simulink library "Lib_LongPRACH"  (R2023b)
settings: Solver=VariableStepAuto  StartTime=0.0  StopTime=10.0  RelTol=1e-3
values from neighbouring files (symbols this model uses):
  prach = waveconfig.PRACH.Config    [hNRPRACHWaveformGenerator.m]
undefined symbols (not defined in the file or in its folder): AdvDSPBChannelOutDisplay, AdvDSPBDMemDisplay, AdvDSPBInDisplay, AdvDSPBOutDisplay, dpoly, dspba, dspba_ChannelInVis, dspba_ChannelOutVis, dspba_internal_get_channel_ports, evalAionMaskParam, latency, latencyCorrection, NTxAnts, primtype, UseDontCare, value
libraries: DSPBAPrim x553, DSPBABase x32, DSPBAFilters x24, DSPBAControl x18, DSPBAModelBus x8, DSPBAWaveformSynth x4, DspbAdvFftLibrary x2, DSPBAUtilities x2
(part 1 of 8)
settings Model: Creator=manjukri  LastModifiedBy=5g
settings ModelReferenceCC: EnableRefExpFcnMdlSchedulingChecks=on

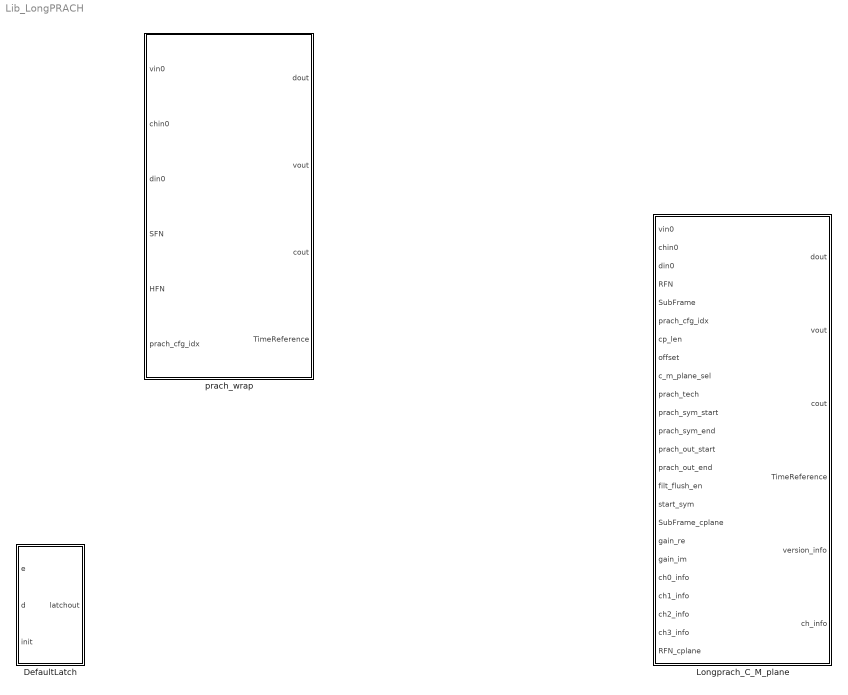
== system Lib_LongPRACH ==
  DefaultLatch : Subsystem
  Longprach_C_M_plane : Subsystem  mask{AxCdelay=60, FFT_frac_scaling=8, gain_out_frac=11}
      mask prompts: AxCdelay "Enter the output delay between antenna(min 60)"; FFT_frac_scaling "FFT output Fractional bits"; gain_out_frac "Gain block output fractional bits"
      mask init:
      | fsmpaths
      | %% 3GPP TS 38.211 V17.2  Table 6.3.3.2-3
      | 
      | Map_5g_LUT1 = [9 9 9 9 9 4 4 9 8 7 6 5 4 3 2 1 1 4 3 2 8 4 3 7 3 6 1 1 zeros(1,512-35) 7 7 7 7 7 2 2 ];
      | Map_5g_LUT2 = [9 9 9 9 9 4 4 9 8 7 6 5 4 3 2 6 6 9 8 7 9 8 4 8 4 7 4 3 zeros(1,512-35) 7 7 7 7 7 2 2 ];
      | Map_5g_LUT3 = [9 9 9 9 9 4 4 9 8 7 6 5 4 3 2 6 6 9 8 7 9 9 9 9 8 8 6 5 zeros(1,512-35) 7 7 7 7 7 2 2 ];
      | Map_5g_LUT4 = [9 9 9 9 9 4 4 9 8 7 6 5 4 3 2 6 6 9 8 7 9 9 9 9 9 9 9 7 zeros(1,512-35) 7 7 7 7 7 2 2 ];
      | Map_5g_LUT5 = [9 9 9 9 9 4 4 9 8 7 6 5 4 3 2 6 6 9 8 7 9 9 9 9 9 9 9 9 zeros(1,512-35) 7 7 7 7 7 2 2 ];
      | 
      | 
      | x_lut = [16,8,4,2,2,2,2,ones(1,512-14),16,8,4,2,2,2,2];
      | y_lut = [1 1 1 0 1 0  1 zeros(1,512-14) 1 1 1 0 1 0 1];
      | 
      | startsym_lut=[ones(1,16) 8 ones(1,512-17)];
  prach_wrap : Subsystem  mask{LongFormat=0, prach_technology=1, AxCdelay=60, PRACH_SCS=1.25, FFT_frac_scaling=12}
      mask prompts: LongFormat "Enter PRACH Long Format"; prach_technology "Enter Technology : 0=4G , 1=5G"; AxCdelay "Enter the output delay between antenna(min 60)"; PRACH_SCS "Enter PRACH subcarrier Spacing (KHz)"; FFT_frac_scaling "FFT output Fractional bits"
      mask init:
      | fsmpaths
      | %% 3GPP TS 38.211 V17.2  Table 6.3.3.2-3
      | 
      | Map_5g_LUT1 = [9 9 9 9 9 4 4 9 8 7 6 5 4 3 2 1 1 4 3 2 8 4 3 7 3 6 1 1 zeros(1,256-28)];
      | Map_5g_LUT2 = [9 9 9 9 9 4 4 9 8 7 6 5 4 3 2 6 6 9 8 7 9 8 4 8 4 7 4 3 zeros(1,256-28)];
      | Map_5g_LUT3 = [9 9 9 9 9 4 4 9 8 7 6 5 4 3 2 6 6 9 8 7 9 9 9 9 8 8 6 5 zeros(1,256-28)];
      | Map_5g_LUT4 = [9 9 9 9 9 4 4 9 8 7 6 5 4 3 2 6 6 9 8 7 9 9 9 9 9 9 9 7 zeros(1,256-28)];
      | Map_5g_LUT5 = [9 9 9 9 9 4 4 9 8 7 6 5 4 3 2 6 6 9 8 7 9 9 9 9 9 9 9 9 zeros(1,256-28)];

== system Lib_LongPRACH/DefaultLatch ==
  e : Inport
  d : Inport  Port=2
  init : Inport  Port=3
  Mux : DSPBAPrim/Mux  primtype=mux  nInputs=evalAionMaskParam(gcb,'value',1)+1  nOutputs=1  omode=Inherit via internal rule  otype=sfix(16)  scale=2^-15  rndmethod=Unbiased  factor=1  satmethod=Symmetric  shift_vec=[0 1 2 -1]  value=2  inPortNames=['s '; 'd0'; 'd1'; 'd2'; 'd3'; 'd4'; 'd5'; 'd6'; 'd7'; 'd8'; 'd9';]  outPortNames=[' ']  dspbaimage=dspba_prim_tall.svg  text=fprintf('%s', primtype);  style=Optimised  visibilities=1032  version=20211007
  Or : DSPBAPrim/Or  primtype=or  nInputs=2  nOutputs=1  omode=Inherit via internal rule  otype=sfix(16)  scale=2^-15  rndmethod=Unbiased  factor=1  satmethod=Symmetric  shift_vec=[0 1 2 -1]  value=0  inPortNames=[' '; ' '; ' '; ' '; ' '; ' '; ' '; ' '; ' '; ' '; ' '; ' '; ' '; ' '; ' '; ' '; ]  outPortNames=[' ']  dspbaimage=dspba_prim.svg  text=fprintf('|');  style=Optimised  visibilities=8+2  version=20211007
  SampleDelay : DSPBAPrim/SampleDelay  primtype=sampdelay  nInputs=1  nOutputs=1  omode=Inherit via internal rule  otype=sfix(16)  scale=2^-15  rndmethod=Unbiased  factor=1  satmethod=Symmetric  shift_vec=[0 1 2 -1]  floatPrecision=float32_m23  value=1  inPortNames=[' '; ' ';]  outPortNames=[' ']  dspbaimage=dspba_prim.svg  text=dpoly(1, eye(1,value+1), 'z')  style=Optimised  visibilities=8 + 2^11 + 2^18 + 2^19  flexible=off  slackgroup=0  augmented=0  version=20211007  advOptions=[]
  latch_0L : DSPBAControl/latch_0L
  latchout : Outport
  wires:
  Or/1 -> SampleDelay/1, Mux/1
  Mux/1 -> latchout/1
  e/1 -> latch_0L/1, Or/1
  SampleDelay/1 -> Or/2
  init/1 -> Mux/2
  latch_0L/1 -> Mux/3
  d/1 -> latch_0L/2

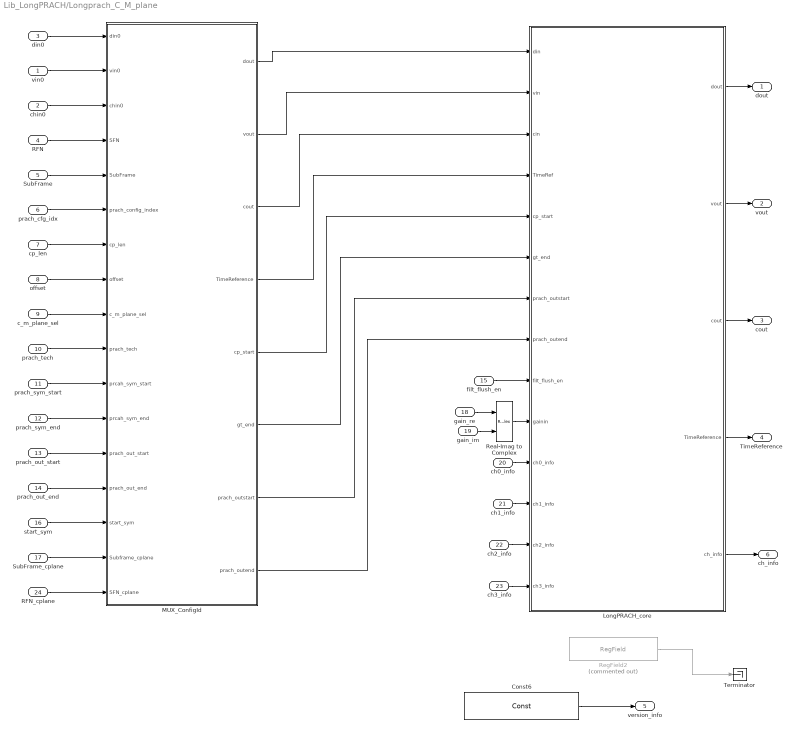
== system Lib_LongPRACH/Longprach_C_M_plane ==
  vin0 : Inport
  chin0 : Inport  Port=2
  din0 : Inport  Port=3
  RFN : Inport  Port=4
  SubFrame : Inport  Port=5
  prach_cfg_idx : Inport  Port=6
  cp_len : Inport  Port=7
  offset : Inport  Port=8
  c_m_plane_sel : Inport  Port=9
  prach_tech : Inport  Port=10
  prach_sym_start : Inport  Port=11
  prach_sym_end : Inport  Port=12
  prach_out_start : Inport  Port=13
  prach_out_end : Inport  Port=14
  filt_flush_en : Inport  Port=15
  start_sym : Inport  Port=16
  SubFrame_cplane : Inport  Port=17
  gain_re : Inport  Port=18
  gain_im : Inport  Port=19
  ch0_info : Inport  Port=20
  ch1_info : Inport  Port=21
  ch2_info : Inport  Port=22
  ch3_info : Inport  Port=23
  RFN_cplane : Inport  Port=24
  Const6 : DSPBAPrim/Const  primtype=const  nInputs=0  nOutputs=1  omode=Specify via dialog  otype=ufix(32)  scale=2^0  rndmethod=Unbiased  factor=1  satmethod=Symmetric  shift_vec=[0 1 2 -1]  value=Version_reg_val  inPortNames=['+'; '+';]  outPortNames=[' ']  dspbaimage=dspba_prim.svg  text=fprintf('%s', num2str(value));  style=Optimised  visibilities=8 + 1024  floatPrecision=float32_m23  warnSaturation=on  version=20211007  SampleTime=inf
  LongPRACH_core : Subsystem
  MUX_ConfigId : Subsystem
  Real-Imag to Complex : RealImagToComplex
  RegField2 : DSPBAModelBus/RegField  Commented=on  reg_name=MMoffset.versionreg  reg_rwmode=Constant  reg_msb=31  reg_lsb=0  reg_mode=Specify via dialog  reg_type=ufix(32)  reg_scale=2^0  reg_init=Version_reg_val  reg_desc=version register  reg_modal=off  reg_desc0=0  reg_desc1=0  reg_desc2=0  reg_desc3=0  reg_desc4=0  reg_desc5=0  reg_desc6=0  reg_desc7=0  reg_addr=4  SampleTime=-1  version=20090407
  Terminator : Terminator
  dout : Outport  VectorParamsAs1DForOutWhenUnconnected=off
  vout : Outport  Port=2  VectorParamsAs1DForOutWhenUnconnected=off
  cout : Outport  Port=3  VectorParamsAs1DForOutWhenUnconnected=off
  TimeReference : Outport  Port=4  VectorParamsAs1DForOutWhenUnconnected=off
  version_info : Outport  Port=5
  ch_info : Outport  Port=6
  wires:
  MUX_ConfigId/7(prach_outstart) -> LongPRACH_core/7(prach_outstart)
  MUX_ConfigId/8(prach_outend) -> LongPRACH_core/8(prach_outend)
  MUX_ConfigId/2(vout) -> LongPRACH_core/2(vin)
  start_sym/1 -> MUX_ConfigId/15(start_sym)
  din0/1 -> MUX_ConfigId/1(din0)
  prach_out_end/1 -> MUX_ConfigId/14(prach_out_end)
  MUX_ConfigId/1(dout) -> LongPRACH_core/1(din)
  prach_out_start/1 -> MUX_ConfigId/13(prach_out_start)
  prach_cfg_idx/1 -> MUX_ConfigId/6(prach_config_index)
  MUX_ConfigId/6(gt_end) -> LongPRACH_core/6(gt_end)
  c_m_plane_sel/1 -> MUX_ConfigId/9(c_m_plane_sel)
  LongPRACH_core/4(TimeReference) -> TimeReference/1
  chin0/1 -> MUX_ConfigId/3(chin0)
  filt_flush_en/1 -> LongPRACH_core/9(filt_flush_en)
  LongPRACH_core/3(cout) -> cout/1
  prach_sym_start/1 -> MUX_ConfigId/11(prcah_sym_start)
  LongPRACH_core/1(dout) -> dout/1
  SubFrame/1 -> MUX_ConfigId/5(SubFrame)
  RFN/1 -> MUX_ConfigId/4(SFN)
  vin0/1 -> MUX_ConfigId/2(vin0)
  LongPRACH_core/2(vout) -> vout/1
  MUX_ConfigId/5(cp_start) -> LongPRACH_core/5(cp_start)
  prach_tech/1 -> MUX_ConfigId/10(prach_tech)
  SubFrame_cplane/1 -> MUX_ConfigId/16(Subframe_cplane)
  MUX_ConfigId/3(cout) -> LongPRACH_core/3(cin)
  MUX_ConfigId/4(TimeReference) -> LongPRACH_core/4(TimeRef)
  offset/1 -> MUX_ConfigId/8(offset)
  prach_sym_end/1 -> MUX_ConfigId/12(prcah_sym_end)
  cp_len/1 -> MUX_ConfigId/7(cp_len)
  Real-Imag to Complex/1 -> LongPRACH_core/10(gainin)
  gain_re/1 -> Real-Imag to Complex/1
  gain_im/1 -> Real-Imag to Complex/2
  RegField2/1 -> Terminator/1
  Const6/1 -> version_info/1
  ch0_info/1 -> LongPRACH_core/11(ch0_info)
  ch2_info/1 -> LongPRACH_core/13(ch2_info)
  ch1_info/1 -> LongPRACH_core/12(ch1_info)
  ch3_info/1 -> LongPRACH_core/14(ch3_info)
  LongPRACH_core/5(ch_info) -> ch_info/1
  RFN_cplane/1 -> MUX_ConfigId/17(SFN_cplane)

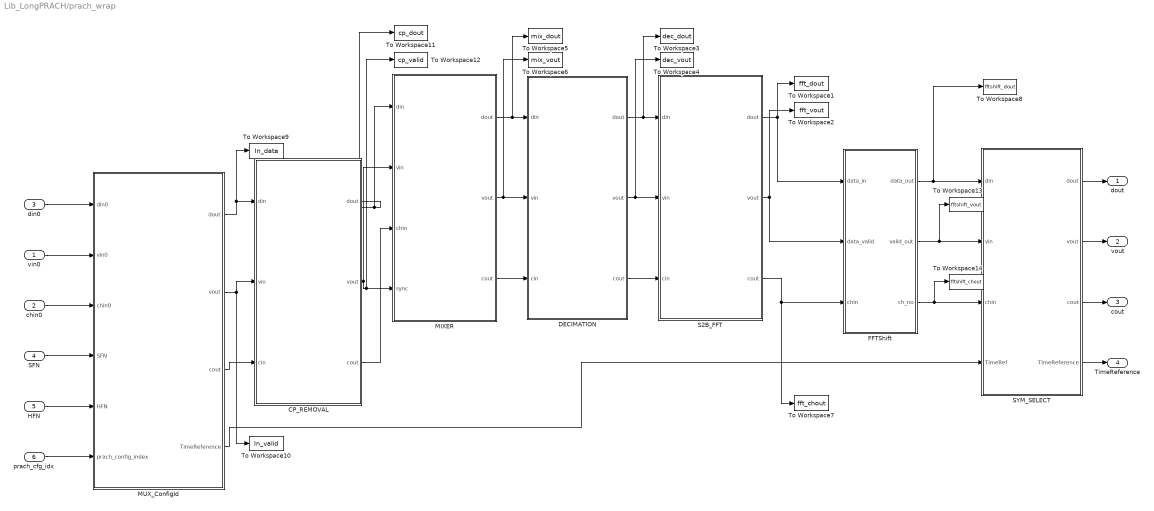
== system Lib_LongPRACH/prach_wrap ==
  vin0 : Inport
  chin0 : Inport  Port=2
  din0 : Inport  Port=3
  SFN : Inport  Port=4
  HFN : Inport  Port=5
  prach_cfg_idx : Inport  Port=6
  CP_REMOVAL : Subsystem
  DECIMATION : Subsystem
  FFTShift : Subsystem
  MIXER : Subsystem
  MUX_ConfigId : Subsystem
  S2B_FFT : Subsystem
  SYM_SELECT : Subsystem
  To Workspace1 : ToWorkspace  VariableName=fft_dout  SampleTime=-1
  To Workspace10 : ToWorkspace  VariableName=In_valid  SampleTime=-1
  To Workspace11 : ToWorkspace  VariableName=cp_dout  SampleTime=-1
  To Workspace12 : ToWorkspace  VariableName=cp_valid  SampleTime=-1
  To Workspace13 : ToWorkspace  VariableName=fftshift_vout  SampleTime=-1
  To Workspace14 : ToWorkspace  VariableName=fftshift_chout  SampleTime=-1
  To Workspace2 : ToWorkspace  VariableName=fft_vout  SampleTime=-1
  To Workspace3 : ToWorkspace  VariableName=dec_dout  SampleTime=-1
  To Workspace4 : ToWorkspace  VariableName=dec_vout  SampleTime=-1
  To Workspace5 : ToWorkspace  VariableName=mix_dout  SampleTime=-1
  To Workspace6 : ToWorkspace  VariableName=mix_vout  SampleTime=-1
  To Workspace7 : ToWorkspace  VariableName=fft_chout  SampleTime=-1
  To Workspace8 : ToWorkspace  VariableName=fftshift_dout  SampleTime=-1
  To Workspace9 : ToWorkspace  VariableName=In_data  SampleTime=-1
  dout : Outport  VectorParamsAs1DForOutWhenUnconnected=off
  vout : Outport  Port=2  VectorParamsAs1DForOutWhenUnconnected=off
  cout : Outport  Port=3  VectorParamsAs1DForOutWhenUnconnected=off
  TimeReference : Outport  Port=4  VectorParamsAs1DForOutWhenUnconnected=off
  wires:
  MUX_ConfigId/1(dout) -> To Workspace9/1, CP_REMOVAL/1(din)
  DECIMATION/1(dout) -> S2B_FFT/1(din), To Workspace3/1
  MIXER/2(vout) -> DECIMATION/2(vin), To Workspace6/1
  MUX_ConfigId/2(vout) -> To Workspace10/1, CP_REMOVAL/2(vin)
  CP_REMOVAL/2(vout) -> To Workspace12/1, MIXER/4(sync), MIXER/2(vin)
  MUX_ConfigId/4(TimeReference) -> SYM_SELECT/4(TimeRef)
  S2B_FFT/3(cout) -> FFTShift/3(chin), To Workspace7/1
  DECIMATION/2(vout) -> S2B_FFT/2(vin), To Workspace4/1
  SYM_SELECT/2(vout) -> vout/1
  S2B_FFT/2(vout) -> FFTShift/2(data_valid), To Workspace2/1
  MIXER/3(cout) -> DECIMATION/3(cin)
  CP_REMOVAL/1(dout) -> To Workspace11/1, MIXER/1(din)
  CP_REMOVAL/3(cout) -> MIXER/3(chin)
  MIXER/1(dout) -> DECIMATION/1(din), To Workspace5/1
  DECIMATION/3(cout) -> S2B_FFT/3(cin)
  SYM_SELECT/3(cout) -> cout/1
  SFN/1 -> MUX_ConfigId/4(SFN)
  HFN/1 -> MUX_ConfigId/5(HFN)
  MUX_ConfigId/3(cout) -> CP_REMOVAL/3(cin)
  din0/1 -> MUX_ConfigId/1(din0)
  prach_cfg_idx/1 -> MUX_ConfigId/6(prach_config_index)
  chin0/1 -> MUX_ConfigId/3(chin0)
  S2B_FFT/1(dout) -> FFTShift/1(data_in), To Workspace1/1
  SYM_SELECT/1(dout) -> dout/1
  SYM_SELECT/4(TimeReference) -> TimeReference/1
  vin0/1 -> MUX_ConfigId/2(vin0)
  FFTShift/1(data_out) -> To Workspace8/1, SYM_SELECT/1(din)
  FFTShift/2(valid_out) -> To Workspace13/1, SYM_SELECT/2(vin)
  FFTShift/3(ch_no) -> To Workspace14/1, SYM_SELECT/3(chin)

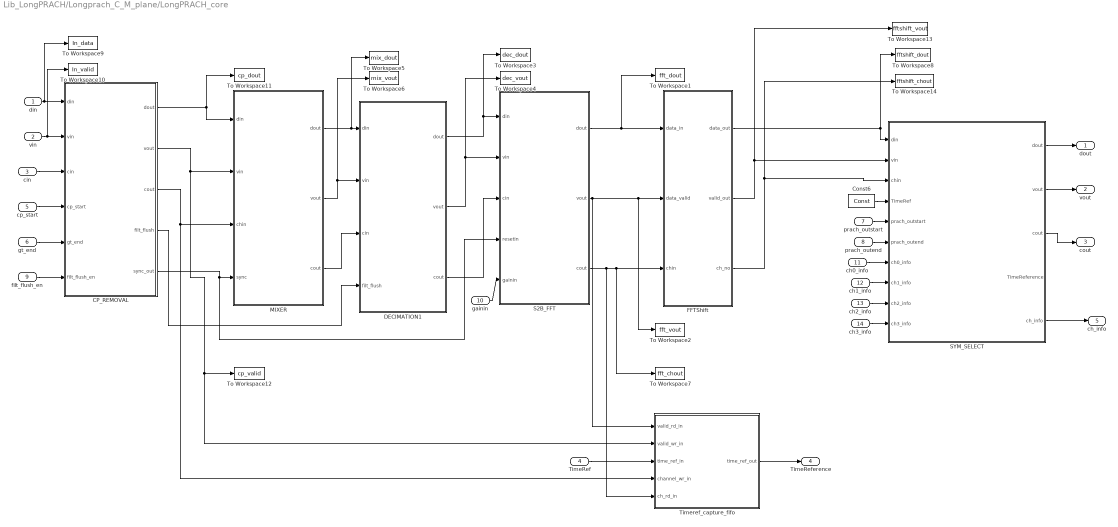
== system Lib_LongPRACH/Longprach_C_M_plane/LongPRACH_core ==
  din : Inport
  vin : Inport  Port=2
  cin : Inport  Port=3
  TimeRef : Inport  Port=4
  cp_start : Inport  Port=5
  gt_end : Inport  Port=6
  prach_outstart : Inport  Port=7
  prach_outend : Inport  Port=8
  filt_flush_en : Inport  Port=9
  gainin : Inport  Port=10
  ch0_info : Inport  Port=11
  ch1_info : Inport  Port=12
  ch2_info : Inport  Port=13
  ch3_info : Inport  Port=14
  CP_REMOVAL : Subsystem
  Const6 : DSPBAPrim/Const  primtype=const  nInputs=0  nOutputs=1  omode=Specify via dialog  otype=ufix(1)  scale=2^0  rndmethod=Unbiased  factor=1  satmethod=Symmetric  shift_vec=[0 1 2 -1]  value=0  inPortNames=['+'; '+';]  outPortNames=[' ']  dspbaimage=dspba_prim.svg  text=fprintf('%s', num2str(value));  style=Optimised  visibilities=8 + 1024  floatPrecision=float32_m23  warnSaturation=on  version=20211007  SampleTime=inf
  DECIMATION1 : Subsystem
  FFTShift : Subsystem
  MIXER : Subsystem
  S2B_FFT : Subsystem
  SYM_SELECT : Subsystem
  Timeref_capture_fifo : Subsystem
  To Workspace1 : ToWorkspace  VariableName=fft_dout  SampleTime=-1
  To Workspace10 : ToWorkspace  VariableName=In_valid  SampleTime=-1
  To Workspace11 : ToWorkspace  VariableName=cp_dout  SampleTime=-1
  To Workspace12 : ToWorkspace  VariableName=cp_valid  SampleTime=-1
  To Workspace13 : ToWorkspace  VariableName=fftshift_vout  SampleTime=-1
  To Workspace14 : ToWorkspace  VariableName=fftshift_chout  SampleTime=-1
  To Workspace2 : ToWorkspace  VariableName=fft_vout  SampleTime=-1
  To Workspace3 : ToWorkspace  VariableName=dec_dout  SampleTime=-1
  To Workspace4 : ToWorkspace  VariableName=dec_vout  SampleTime=-1
  To Workspace5 : ToWorkspace  VariableName=mix_dout  SampleTime=-1
  To Workspace6 : ToWorkspace  VariableName=mix_vout  SampleTime=-1
  To Workspace7 : ToWorkspace  VariableName=fft_chout  SampleTime=-1
  To Workspace8 : ToWorkspace  VariableName=fftshift_dout  SampleTime=-1
  To Workspace9 : ToWorkspace  VariableName=In_data  SampleTime=-1
  dout : Outport
  vout : Outport  Port=2
  cout : Outport  Port=3
  TimeReference : Outport  Port=4
  ch_info : Outport  Port=5
  wires:
  SYM_SELECT/3(cout) -> cout/1
  SYM_SELECT/2(vout) -> vout/1
  SYM_SELECT/1(dout) -> dout/1
  prach_outend/1 -> SYM_SELECT/6(prach_outend)
  prach_outstart/1 -> SYM_SELECT/5(prach_outstart)
  Const6/1 -> SYM_SELECT/4(TimeRef)
  FFTShift/3(ch_no) -> To Workspace14/1, SYM_SELECT/3(chin)
  FFTShift/1(data_out) -> To Workspace8/1, SYM_SELECT/1(din)
  TimeRef/1 -> Timeref_capture_fifo/3(time_ref_in)
  S2B_FFT/3(cout) -> FFTShift/3(chin), To Workspace7/1, Timeref_capture_fifo/5(ch_rd_in)
  S2B_FFT/1(dout) -> FFTShift/1(data_in), To Workspace1/1
  DECIMATION1/3(cout) -> S2B_FFT/3(cin)
  CP_REMOVAL/3(cout) -> Timeref_capture_fifo/4(channel_wr_in), MIXER/3(chin)
  cin/1 -> CP_REMOVAL/3(cin)
  FFTShift/2(valid_out) -> To Workspace13/1, SYM_SELECT/2(vin)
  vin/1 -> CP_REMOVAL/2(vin), To Workspace10/1
  CP_REMOVAL/2(vout) -> Timeref_capture_fifo/2(valid_wr_in), To Workspace12/1, MIXER/2(vin)
  cp_start/1 -> CP_REMOVAL/4(cp_start)
  MIXER/2(vout) -> DECIMATION1/2(vin), To Workspace6/1
  CP_REMOVAL/1(dout) -> MIXER/1(din), To Workspace11/1
  MIXER/1(dout) -> DECIMATION1/1(din), To Workspace5/1
  DECIMATION1/1(dout) -> S2B_FFT/1(din), To Workspace3/1
  Timeref_capture_fifo/1(time_ref_out) -> TimeReference/1
  MIXER/3(cout) -> DECIMATION1/3(cin)
  S2B_FFT/2(vout) -> FFTShift/2(data_valid), To Workspace2/1, Timeref_capture_fifo/1(valid_rd_in)
  din/1 -> To Workspace9/1, CP_REMOVAL/1(din)
  DECIMATION1/2(vout) -> S2B_FFT/2(vin), To Workspace4/1
  CP_REMOVAL/4(filt_flush) -> DECIMATION1/4(filt_flush)
  filt_flush_en/1 -> CP_REMOVAL/6(filt_flush_en)
  gt_end/1 -> CP_REMOVAL/5(gt_end)
  CP_REMOVAL/5(sync_out) -> S2B_FFT/4(resetin), MIXER/4(sync)
  gainin/1 -> S2B_FFT/5(gainin)
  ch0_info/1 -> SYM_SELECT/7(ch0_info)
  ch1_info/1 -> SYM_SELECT/8(ch1_info)
  ch2_info/1 -> SYM_SELECT/9(ch2_info)
  ch3_info/1 -> SYM_SELECT/10(ch3_info)
  SYM_SELECT/5(ch_info) -> ch_info/1

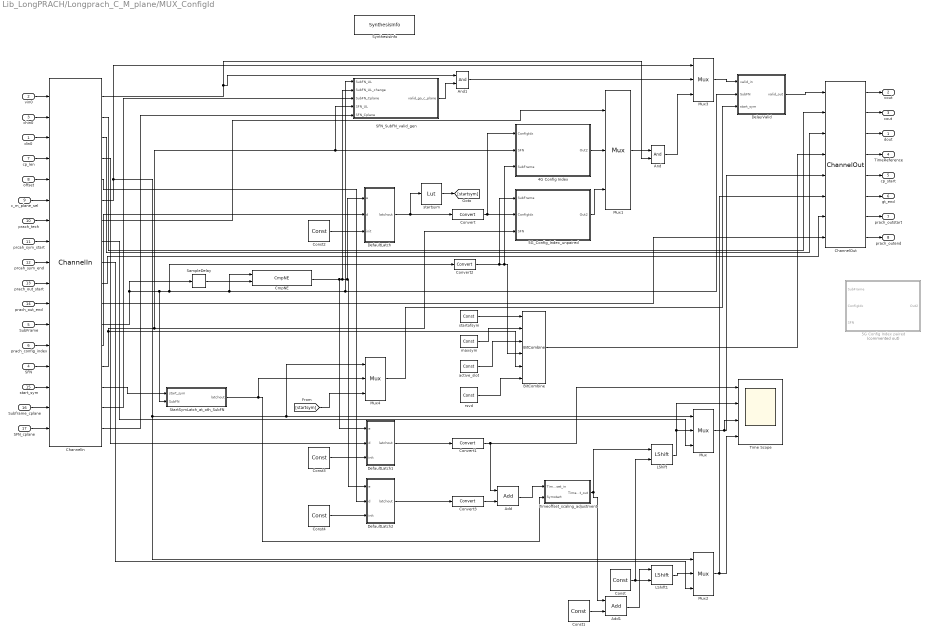
== system Lib_LongPRACH/Longprach_C_M_plane/MUX_ConfigId ==
  din0 : Inport
  vin0 : Inport  Port=2  OutDataTypeStr=boolean
  chin0 : Inport  Port=3  OutDataTypeStr=uint8
  SFN : Inport  Port=4
  SubFrame : Inport  Port=5
  prach_config_index : Inport  Port=6
  cp_len : Inport  Port=7
  offset : Inport  Port=8
  c_m_plane_sel : Inport  Port=9
  prach_tech : Inport  Port=10
  prcah_sym_start : Inport  Port=11
  prcah_sym_end : Inport  Port=12
  prach_out_start : Inport  Port=13
  prach_out_end : Inport  Port=14
  start_sym : Inport  Port=15
  Subframe_cplane : Inport  Port=16
  SFN_cplane : Inport  Port=17
  4G Config Index : Subsystem
  5G Config Index paired : Subsystem  Commented=on
  5G_Config_Index_unpaired : Subsystem
  Add : DSPBAPrim/Add  primtype=add  nInputs=evalAionMaskParam(gcb,'value',1)  nOutputs=1  omode=Inherit via internal rule with word growth  otype=sfix(16)  scale=2^-15  rndmethod=Unbiased  factor=1  satmethod=Symmetric  shift_vec=[0 1 2 -1]  value=2  inPortNames=[' '; ' ';]  outPortNames=[' ']  dspbaimage=dspba_prim.svg  text=fprintf('+');  style=Optimised  visibilities=1032+2^17+2^18+2^19  genFPC=off  floatRounding=correct  advOptions=[]  version=20211007
  Add1 : DSPBAPrim/Add  primtype=add  nInputs=evalAionMaskParam(gcb,'value',1)  nOutputs=1  omode=Inherit via internal rule with word growth  otype=sfix(16)  scale=2^-15  rndmethod=Unbiased  factor=1  satmethod=Symmetric  shift_vec=[0 1 2 -1]  value=2  inPortNames=[' '; ' ';]  outPortNames=[' ']  dspbaimage=dspba_prim.svg  text=fprintf('+');  style=Optimised  visibilities=1032+2^17+2^18+2^19  genFPC=off  floatRounding=correct  advOptions=[]  version=20211007
  And : DSPBAPrim/And  primtype=and  nInputs=2  nOutputs=1  omode=Inherit via internal rule  otype=sfix(16)  scale=2^-15  rndmethod=Unbiased  factor=1  satmethod=Symmetric  shift_vec=[0 1 2 -1]  value=0  inPortNames=[' '; ' '; ' '; ' '; ' '; ' '; ' '; ' '; ' '; ' '; ' '; ' '; ' '; ' '; ' '; ' '; ]  outPortNames=[' ']  dspbaimage=dspba_prim.svg  text=fprintf('&');  style=Optimised  visibilities=8+2  version=20211007
  And1 : DSPBAPrim/And  primtype=and  nInputs=2  nOutputs=1  omode=Inherit via internal rule  otype=sfix(16)  scale=2^-15  rndmethod=Unbiased  factor=1  satmethod=Symmetric  shift_vec=[0 1 2 -1]  value=0  inPortNames=[' '; ' '; ' '; ' '; ' '; ' '; ' '; ' '; ' '; ' '; ' '; ' '; ' '; ' '; ' '; ' '; ]  outPortNames=[' ']  dspbaimage=dspba_prim.svg  text=fprintf('&');  style=Optimised  visibilities=8+2  version=20211007
  BitCombine : DSPBAPrim/BitCombine  primtype=bitcombine  nInputs=6  nOutputs=1  omode=Inherit via internal rule  otype=sfix(16)  scale=2^-15  rndmethod=Unbiased  factor=1  satmethod=Symmetric  shift_vec=[0 1 2 -1]  value=0  inPortNames=['l'; 'h';]  outPortNames=[' ']  dspbaimage=dspba_prim.svg  text=fprintf('[h,l]');  style=Optimised  visibilities=8+2  version=20211007
  ChannelIn : DSPBAPrim/ChannelIn  primtype=channelin  nInputs=dspba_internal_get_channel_ports(gcb)  nOutputs=dspba_internal_get_channel_ports(gcb)  omode=Inherit via internal rule  otype=sfix(16)  scale=2^-15  rndmethod=Unbiased  factor=1  satmethod=Symmetric  shift_vec=[0 1 2 -1]  value=15  inPortNames=['v'; 'c'; '0'; '1'; '2'; '3'; '4'; '5'; '6'; '7'; '8'; '9'; 'A'; 'B'; 'D'; 'E'; 'F'; 'G'; 'H'; 'I'; 'J'; 'K'; 'L'; 'M'; 'N'; 'O'; 'P'; 'Q'; 'R'; 'S'; 'T'; 'U'; 'W'; 'X'; 'Y'; 'Z']  outPortNames=['v'; 'c'; '0'; '1'; '2'; '3'; '4'; '5'; '6'; '7'; '8'; '9'; 'A'; 'B'; 'D'; 'E'; 'F'; 'G'; 'H'; 'I'; 'J'; 'K'; 'L'; 'M'; 'N'; 'O'; 'P'; 'Q'; 'R'; 'S'; 'T'; 'U'; 'W'; 'X'; 'Y'; 'Z']  dspbaimage=dspba_prim_channel_tall.svg  text=fprintf('In');  style=Optimised  dataSignals=15  foldingEnabled=off  channels=1  sampleRate=200  packetBeginPresent=off  packetBeginEnabled=off  visibilities=dspba_ChannelInVis(gcb)  latencyCorrection=0  scheduleOrigin=on  version=20211214
  ChannelOut : DSPBAPrim/ChannelOut  primtype=channelout  nInputs=dspba_internal_get_channel_ports(gcb)  nOutputs=dspba_internal_get_channel_ports(gcb)  omode=Inherit via internal rule  otype=sfix(16)  scale=2^-15  rndmethod=Unbiased  factor=1  satmethod=Symmetric  shift_vec=[0 1 2 -1]  value=6  inPortNames=['v'; 'c'; '0'; '1'; '2'; '3'; '4'; '5'; '6'; '7'; '8'; '9'; 'A'; 'B'; 'D'; 'E'; 'F'; 'G'; 'H'; 'I'; 'J'; 'K'; 'L'; 'M'; 'N'; 'O'; 'P'; 'Q'; 'R'; 'S'; 'T'; 'U'; 'W'; 'X'; 'Y'; 'Z']  outPortNames=['v'; 'c'; '0'; '1'; '2'; '3'; '4'; '5'; '6'; '7'; '8'; '9'; 'A'; 'B'; 'D'; 'E'; 'F'; 'G'; 'H'; 'I'; 'J'; 'K'; 'L'; 'M'; 'N'; 'O'; 'P'; 'Q'; 'R'; 'S'; 'T'; 'U'; 'W'; 'X'; 'Y'; 'Z']  dspbaimage=dspba_prim_channel_tall.svg  text=fprintf('Out%s', AdvDSPBChannelOutDisplay(latency));  style=Optimised  dataSignals=6  foldingEnabled=off  channels=1  sampleRate=200  packetBeginPresent=off  packetBeginEnabled=off  visibilities=dspba_ChannelOutVis(gcb)  latency=21  latencyCorrection=0  version=20211214
  CmpNE : DSPBAPrim/CmpNE  primtype=cmpne  nInputs=2  nOutputs=1  omode=boolean  otype=sfix(16)  scale=2^-15  rndmethod=Unbiased  factor=1  satmethod=Symmetric  shift_vec=[0 1 2 -1]  value=0  inPortNames=[' '; ' ';]  outPortNames=[' ']  dspbaimage=dspba_prim.svg  text=fprintf('~=');  style=Optimised  visibilities=0  advOptions=[]  version=20211007
  Const : DSPBAPrim/Const  primtype=const  nInputs=0  nOutputs=1  omode=Inherit via internal rule  otype=sfix(16)  scale=2^-15  rndmethod=Unbiased  factor=1  satmethod=Symmetric  shift_vec=[0 1 2 -1]  value=2*log2(NTxAnts)  inPortNames=['+'; '+';]  outPortNames=[' ']  dspbaimage=dspba_prim.svg  text=fprintf('%s', num2str(value));  style=Optimised  visibilities=8 + 1024 + 2^18 + 2^20  floatPrecision=float32_m23  warnSaturation=on  version=20211007  SampleTime=inf
  Const1 : DSPBAPrim/Const  primtype=const  nInputs=0  nOutputs=1  omode=Inherit via internal rule  otype=sfix(16)  scale=2^-15  rndmethod=Unbiased  factor=1  satmethod=Symmetric  shift_vec=[0 1 2 -1]  value=prach.seqlength/4  inPortNames=['+'; '+';]  outPortNames=[' ']  dspbaimage=dspba_prim.svg  text=fprintf('%s', num2str(value));  style=Optimised  visibilities=8 + 1024 + 2^18 + 2^20  floatPrecision=float32_m23  warnSaturation=on  version=20211007  SampleTime=inf
  Const2 : DSPBAPrim/Const  primtype=const  nInputs=0  nOutputs=1  omode=Specify via dialog  otype=ufix(16)  scale=0  rndmethod=Unbiased  factor=1  satmethod=Symmetric  shift_vec=[0 1 2 -1]  value=27  inPortNames=['+'; '+';]  outPortNames=[' ']  dspbaimage=dspba_prim.svg  text=fprintf('%s', num2str(value));  style=Optimised  visibilities=8 + 1024 + 2^18 + 2^20  floatPrecision=float32_m23  warnSaturation=on  version=20211007  SampleTime=inf
  Const3 : DSPBAPrim/Const  primtype=const  nInputs=0  nOutputs=1  omode=Specify via dialog  otype=ufix(21)  scale=0  rndmethod=Unbiased  factor=1  satmethod=Symmetric  shift_vec=[0 1 2 -1]  value=0  inPortNames=['+'; '+';]  outPortNames=[' ']  dspbaimage=dspba_prim.svg  text=fprintf('%s', num2str(value));  style=Optimised  visibilities=8 + 1024 + 2^18 + 2^20  floatPrecision=float32_m23  warnSaturation=on  version=20211007  SampleTime=inf
  Const4 : DSPBAPrim/Const  primtype=const  nInputs=0  nOutputs=1  omode=Specify via dialog  otype=ufix(21)  scale=0  rndmethod=Unbiased  factor=1  satmethod=Symmetric  shift_vec=[0 1 2 -1]  value=3168  inPortNames=['+'; '+';]  outPortNames=[' ']  dspbaimage=dspba_prim.svg  text=fprintf('%s', num2str(value));  style=Optimised  visibilities=8 + 1024 + 2^18 + 2^20  floatPrecision=float32_m23  warnSaturation=on  version=20211007  SampleTime=inf
  Convert : DSPBAPrim/Convert  primtype=convert  nInputs=1  nOutputs=1  omode=Specify via dialog  otype=ufix(16)  scale=0  rndmethod=Unbiased  factor=1  satmethod=None  shift_vec=[0 1 2 -1]  value=round([0:255]/17)  inPortNames=[' '; ' ';]  outPortNames=[' '; 'c']  dspbaimage=dspba_prim_wide.svg  text=fprintf('convert');  style=Optimised  visibilities=8+64+256+2^17  clipdetect=off  floatPrecision=float32_m23  advOptions=[]  version=20211007
  Convert1 : DSPBAPrim/Convert  primtype=convert  nInputs=1  nOutputs=1  omode=Specify via dialog  otype=ufix(21)  scale=0  rndmethod=Unbiased  factor=1  satmethod=None  shift_vec=[0 1 2 -1]  value=round([0:255]/17)  inPortNames=[' '; ' ';]  outPortNames=[' '; 'c']  dspbaimage=dspba_prim_wide.svg  text=fprintf('convert');  style=Optimised  visibilities=8+64+256+2^17  clipdetect=off  floatPrecision=float32_m23  advOptions=[]  version=20211007
  Convert2 : DSPBAPrim/Convert  primtype=convert  nInputs=1  nOutputs=1  omode=Specify via dialog  otype=uint(8)  scale=2^0  rndmethod=Truncate  factor=1  satmethod=None  shift_vec=[0 1 2 -1]  value=round([0:255]/17)  inPortNames=[' '; ' ';]  outPortNames=[' '; 'c']  dspbaimage=dspba_prim_wide.svg  text=fprintf('convert');  style=Optimised  visibilities=8+64+256+2^17  clipdetect=off  floatPrecision=float32_m23  advOptions=[]  version=20211007
  Convert3 : DSPBAPrim/Convert  primtype=convert  nInputs=1  nOutputs=1  omode=Specify via dialog  otype=ufix(21)  scale=0  rndmethod=Unbiased  factor=1  satmethod=None  shift_vec=[0 1 2 -1]  value=round([0:255]/17)  inPortNames=[' '; ' ';]  outPortNames=[' '; 'c']  dspbaimage=dspba_prim_wide.svg  text=fprintf('convert');  style=Optimised  visibilities=8+64+256+2^17  clipdetect=off  floatPrecision=float32_m23  advOptions=[]  version=20211007
  DefaultLatch : Subsystem
  DefaultLatch1 : Subsystem
  DefaultLatch2 : Subsystem
  DelayValid : Subsystem
  LShift : DSPBAPrim/LShift  primtype=lshift  nInputs=2  nOutputs=1  omode=Inherit via internal rule  otype=sfix(16)  scale=2^-15  rndmethod=Unbiased  factor=1  satmethod=Symmetric  shift_vec=[0 1 2 -1]  value=0  inPortNames=['a'; 'b';]  outPortNames=[' ']  dspbaimage=dspba_prim.svg  text=fprintf('a << b');  style=Optimised  visibilities=8  version=20211007
  LShift1 : DSPBAPrim/LShift  primtype=lshift  nInputs=2  nOutputs=1  omode=Inherit via internal rule  otype=sfix(16)  scale=2^-15  rndmethod=Unbiased  factor=1  satmethod=Symmetric  shift_vec=[0 1 2 -1]  value=0  inPortNames=['a'; 'b';]  outPortNames=[' ']  dspbaimage=dspba_prim.svg  text=fprintf('a << b');  style=Optimised  visibilities=8  version=20211007
  Mux{,1..4} (5 alike) : DSPBAPrim/Mux  primtype=mux  nInputs=evalAionMaskParam(gcb,'value',1)+1  nOutputs=1  omode=Inherit via internal rule  otype=sfix(16)  scale=2^-15  rndmethod=Unbiased  factor=1  satmethod=Symmetric  shift_vec=[0 1 2 -1]  value=2  inPortNames=['s '; 'd0'; 'd1'; 'd2'; 'd3'; 'd4'; 'd5'; 'd6'; 'd7'; 'd8'; 'd9';]  outPortNames=[' ']  dspbaimage=dspba_prim_tall.svg  text=fprintf('%s', primtype);  style=Optimised  visibilities=1032  version=20211007
  SFN_SubFN_valid_gen : Subsystem
  SampleDelay : DSPBAPrim/SampleDelay  primtype=sampdelay  nInputs=1  nOutputs=1  omode=Inherit via internal rule  otype=sfix(16)  scale=2^-15  rndmethod=Unbiased  factor=1  satmethod=Symmetric  shift_vec=[0 1 2 -1]  floatPrecision=float32_m23  value=1  inPortNames=[' '; ' ';]  outPortNames=[' ']  dspbaimage=dspba_prim.svg  text=dpoly(1, eye(1,value+1), 'z')  style=Optimised  visibilities=8 + 2^11 + 2^18 + 2^19  flexible=off  slackgroup=0  augmented=0  version=20211007  advOptions=[]
  StartSymLatch_at_oth_SubFN : Subsystem
  SynthesisInfo : DSPBAPrim/SynthesisInfo  primtype=synthinfo  nInputs=0  nOutputs=0  omode=Inherit via internal rule  otype=sfix(16)  scale=2^-15  rndmethod=Truncate  factor=1  satmethod=Symmetric  shift_vec=[0 1 2 -1]  value=99  inPortNames=[' '; ' ';]  outPortNames=[' ']  dspbaimage=dspba_prim_ctrl.jpg  text=fprintf('Style=%s', style);  style=Scheduled  visibilities=2^17+2^18+2^19+2^20+2^21+2^22+2^23+2^24  constraintPair=None  constraintRelation=>  constraintLimit=2  modelRefSign=+  modelRef=''  showSchedule=off  simulationMode=Use Global Value  resetMinimization=Conditional - On for ChannelIn/Out only  version=20220106
  Time Scope : Scope  NumInputPorts=4
  Timeoffset_scaling_adjustment : Subsystem
  active_slot : DSPBAPrim/Const  primtype=const  nInputs=0  nOutputs=1  omode=boolean  otype=ufix(4)  scale=2^0  rndmethod=Unbiased  factor=1  satmethod=Symmetric  shift_vec=[0 1 2 -1]  value=0  inPortNames=['+'; '+';]  outPortNames=[' ']  dspbaimage=dspba_prim.svg  text=fprintf('%s', num2str(value));  style=Optimised  visibilities=8 + 1024 + 2^18 + 2^20  floatPrecision=float32_m23  warnSaturation=on  version=20211007  SampleTime=inf
  maxsym : DSPBAPrim/Const  primtype=const  nInputs=0  nOutputs=1  omode=Specify via dialog  otype=ufix(4)  scale=2^0  rndmethod=Unbiased  factor=1  satmethod=Symmetric  shift_vec=[0 1 2 -1]  value=1  inPortNames=['+'; '+';]  outPortNames=[' ']  dspbaimage=dspba_prim.svg  text=fprintf('%s', num2str(value));  style=Optimised  visibilities=8 + 1024 + 2^18 + 2^20  floatPrecision=float32_m23  warnSaturation=on  version=20211007  SampleTime=inf
  rsvd : DSPBAPrim/Const  primtype=const  nInputs=0  nOutputs=1  omode=Specify via dialog  otype=ufix(3)  scale=2^0  rndmethod=Unbiased  factor=1  satmethod=Symmetric  shift_vec=[0 1 2 -1]  value=0  inPortNames=['+'; '+';]  outPortNames=[' ']  dspbaimage=dspba_prim.svg  text=fprintf('%s', num2str(value));  style=Optimised  visibilities=8 + 1024 + 2^18 + 2^20  floatPrecision=float32_m23  warnSaturation=on  version=20211007  SampleTime=inf
  startofsym : DSPBAPrim/Const  primtype=const  nInputs=0  nOutputs=1  omode=Specify via dialog  otype=ufix(4)  scale=2^0  rndmethod=Unbiased  factor=1  satmethod=Symmetric  shift_vec=[0 1 2 -1]  value=0  inPortNames=['+'; '+';]  outPortNames=[' ']  dspbaimage=dspba_prim.svg  text=fprintf('%s', num2str(value));  style=Optimised  visibilities=8 + 1024 + 2^18 + 2^20  floatPrecision=float32_m23  warnSaturation=on  version=20211007  SampleTime=inf
  startsym : DSPBAPrim/Lut  primtype=lut  nInputs=1  nOutputs=1  omode=Inherit via internal rule  otype=sfix(16)  scale=2^-15  rndmethod=Unbiased  factor=1  satmethod=Symmetric  shift_vec=[0 1 2 -1]  value=startsym_lut  inPortNames=[' '; ' ';]  outPortNames=[' ']  dspbaimage=dspba_prim.svg  text=fprintf('LUT');  style=Optimised  visibilities=8 + 1024  floatPrecision=float32_m23  version=20211007
  dout : Outport  VectorParamsAs1DForOutWhenUnconnected=off
  vout : Outport  Port=2  VectorParamsAs1DForOutWhenUnconnected=off
  cout : Outport  Port=3  VectorParamsAs1DForOutWhenUnconnected=off
  TimeReference : Outport  Port=4  VectorParamsAs1DForOutWhenUnconnected=off
  cp_start : Outport  Port=5
  gt_end : Outport  Port=6
  prach_outstart : Outport  Port=7
  prach_outend : Outport  Port=8
  wires:
  Const/1 -> LShift/2, LShift1/2
  Convert2/1 -> BitCombine/4, 4G Config Index/3(SubFrame), 5G_Config_Index_unpaired/1(SubFrame)
  ChannelIn/6 -> Mux2/1, Mux4/1, Mux/1, Mux3/1
  ChannelIn/12 -> SFN_SubFN_valid_gen/1(SubFN_UL), DelayValid/2(SubFN), CmpNE/1, Convert2/1, StartSymLatch_at_oth_SubFN/2(SubFN), SampleDelay/1
  Convert/1 -> 5G_Config_Index_unpaired/2(ConfigIdx), 4G Config Index/1(ConfigIdx)
  ChannelIn/14 -> 5G_Config_Index_unpaired/3(SFN), 4G Config Index/2(SFN), SFN_SubFN_valid_gen/4(SFN_UL), BitCombine/5
  ChannelIn/1 -> And/2, And1/1
  ChannelOut/3 -> dout/1
  ChannelIn/15 -> StartSymLatch_at_oth_SubFN/1(start_sym)
  prach_tech/1 -> ChannelIn/7
  ChannelOut/1 -> vout/1
  ChannelIn/5 -> DefaultLatch2/2(d)
  SFN_SubFN_valid_gen/1(valid_go_c_plane) -> And1/2
  Mux2/1 -> ChannelOut/6, Time Scope/4
  ChannelOut/6 -> gt_end/1
  c_m_plane_sel/1 -> ChannelIn/6
  cp_len/1 -> ChannelIn/4
  startofsym/1 -> BitCombine/1
  Const4/1 -> DefaultLatch2/3(init)
  Convert1/1 -> Time Scope/1, Add/1
  Convert3/1 -> Add/2
  5G_Config_Index_unpaired/1(Out2) -> Mux1/3
  LShift1/1 -> Mux2/2
  4G Config Index/1(Out2) -> Mux1/2
  CmpNE/1 -> DefaultLatch/1(e), DefaultLatch2/1(e), SFN_SubFN_valid_gen/2(SubFN_UL_change), DefaultLatch1/1(e)
  SFN/1 -> ChannelIn/14
  din0/1 -> ChannelIn/3
  StartSymLatch_at_oth_SubFN/1(latchout) -> Mux4/2, Timeoffset_scaling_adjustment/2(Symstart)
  ChannelIn/13 -> DefaultLatch/2(d)
  ChannelIn/10 -> ChannelOut/7
  ChannelOut/8 -> prach_outend/1
  Mux3/1 -> DelayValid/1(valid_in)
  Subframe_cplane/1 -> ChannelIn/16
  SubFrame/1 -> ChannelIn/12
  start_sym/1 -> ChannelIn/15
  And/1 -> Mux3/3
  ChannelIn/16 -> SFN_SubFN_valid_gen/3("SubFN_Cplane ")
  chin0/1 -> ChannelIn/2
  DefaultLatch2/1(latchout) -> Convert3/1
  Timeoffset_scaling_adjustment/1(Timeoffset_out) -> Add1/1, LShift/1
  ChannelIn/8 -> Mux/3
  ChannelIn/3 -> ChannelOut/3
  DefaultLatch1/1(latchout) -> Convert1/1
  And1/1 -> Mux3/2
  ChannelIn/11 -> ChannelOut/8
  DelayValid/1(valid_out) -> ChannelOut/1
  ChannelIn/9 -> Mux2/3
  prcah_sym_start/1 -> ChannelIn/8
  Const1/1 -> Add1/2
  DefaultLatch/1(latchout) -> startsym/1, Convert/1
  Mux/1 -> ChannelOut/5, Time Scope/3
  BitCombine/1 -> ChannelOut/4
  ChannelIn/7 -> Mux1/1
  maxsym/1 -> BitCombine/2
  ChannelOut/7 -> prach_outstart/1
  Const2/1 -> DefaultLatch/3(init)
  ChannelIn/2 -> ChannelOut/2
  LShift/1 -> Time Scope/2, Mux/2
  ChannelOut/2 -> cout/1
  SampleDelay/1 -> CmpNE/2
  prach_out_start/1 -> ChannelIn/10
  ChannelOut/5 -> cp_start/1
  rsvd/1 -> BitCombine/6
  ChannelOut/4 -> TimeReference/1
  prach_config_index/1 -> ChannelIn/13
  offset/1 -> ChannelIn/5
  prcah_sym_end/1 -> ChannelIn/9
  Mux1/1 -> And/1
  prach_out_end/1 -> ChannelIn/11
  vin0/1 -> ChannelIn/1
  Const3/1 -> DefaultLatch1/3(init)
  Add1/1 -> LShift1/1
  active_slot/1 -> BitCombine/3
  ChannelIn/4 -> DefaultLatch1/2(d)
  Add/1 -> Timeoffset_scaling_adjustment/1(Timeoffset_in)
  Mux4/1 -> DelayValid/3(start_sym)
  startsym/1 -> [startsym]
  [startsym] -> Mux4/3
  SFN_cplane/1 -> ChannelIn/17
  ChannelIn/17 -> SFN_SubFN_valid_gen/5(SFN_Cplane)

== system Lib_LongPRACH/prach_wrap/CP_REMOVAL ==
  din : Inport
  vin : Inport  Port=2
  cin : Inport  Port=3
  RegField3 : DSPBAModelBus/RegField  reg_name=MMoffset.prach_symb_start_ch1  reg_rwmode=Read/Write  reg_msb=31  reg_lsb=0  reg_mode=Specify via dialog  reg_type=uint(32)  reg_scale=2^0  reg_init=prach.symStart  reg_desc=PRACH Sym start Register  reg_modal=off  reg_desc0=0  reg_desc1=0  reg_desc2=0  reg_desc3=0  reg_desc4=0  reg_desc5=0  reg_desc6=0  reg_desc7=0  SampleTime=-1  version=20090407
  RegField4 : DSPBAModelBus/RegField  reg_name=MMoffset.prach_symb_end_ch1  reg_rwmode=Read/Write  reg_msb=31  reg_lsb=0  reg_mode=Specify via dialog  reg_type=uint(32)  reg_scale=2^0  reg_init=prach.symEnd  reg_desc=PRACH Sym end Register  reg_modal=off  reg_desc0=0  reg_desc1=0  reg_desc2=0  reg_desc3=0  reg_desc4=0  reg_desc5=0  reg_desc6=0  reg_desc7=0  SampleTime=-1  version=20090407
  RemoveCP5 : Subsystem
  dout : Outport  VectorParamsAs1DForOutWhenUnconnected=off
  vout : Outport  Port=2  VectorParamsAs1DForOutWhenUnconnected=off
  cout : Outport  Port=3  VectorParamsAs1DForOutWhenUnconnected=off
  wires:
  vin/1 -> RemoveCP5/1(vin)
  cin/1 -> RemoveCP5/2(chin)
  RegField4/1 -> RemoveCP5/5(din2)
  RegField3/1 -> RemoveCP5/4(din1)
  din/1 -> RemoveCP5/3(din)
  RemoveCP5/1(vout) -> vout/1
  RemoveCP5/2(cout) -> cout/1
  RemoveCP5/3(dout) -> dout/1

== system Lib_LongPRACH/prach_wrap/DECIMATION ==
  din : Inport
  vin : Inport  Port=2
  cin : Inport  Port=3
  Filt_DEC_by_2_stage2 : Subsystem
  Filt_DEC_by_2_stage3 : Subsystem
  Filt_DEC_by_2_stage4 : Subsystem
  Filt_DEC_by_2_stage5 : Subsystem
  Filt_DEC_by_2_stage6 : Subsystem
  Filt_DEC_by_3_stage1 : Subsystem
  dout : Outport  VectorParamsAs1DForOutWhenUnconnected=off
  vout : Outport  Port=2  VectorParamsAs1DForOutWhenUnconnected=off
  cout : Outport  Port=3  VectorParamsAs1DForOutWhenUnconnected=off
  wires:
  Filt_DEC_by_2_stage2/2(vout) -> Filt_DEC_by_2_stage3/2(vin)
  Filt_DEC_by_2_stage2/1(dout) -> Filt_DEC_by_2_stage3/1(din)
  Filt_DEC_by_3_stage1/3(cout) -> Filt_DEC_by_2_stage2/3(cin)
  cin/1 -> Filt_DEC_by_3_stage1/3(cin)
  din/1 -> Filt_DEC_by_3_stage1/1(din)
  Filt_DEC_by_2_stage2/3(cout) -> Filt_DEC_by_2_stage3/3(cin)
  Filt_DEC_by_3_stage1/2(vout) -> Filt_DEC_by_2_stage2/2(vin)
  Filt_DEC_by_3_stage1/1(dout) -> Filt_DEC_by_2_stage2/1(din)
  vin/1 -> Filt_DEC_by_3_stage1/2(vin)
  Filt_DEC_by_2_stage6/1(dout) -> dout/1
  Filt_DEC_by_2_stage6/2(vout) -> vout/1
  Filt_DEC_by_2_stage6/3(cout) -> cout/1
  Filt_DEC_by_2_stage3/1(dout) -> Filt_DEC_by_2_stage4/1(din)
  Filt_DEC_by_2_stage3/2(vout) -> Filt_DEC_by_2_stage4/2(vin)
  Filt_DEC_by_2_stage3/3(cout) -> Filt_DEC_by_2_stage4/3(cin)
  Filt_DEC_by_2_stage4/1(dout) -> Filt_DEC_by_2_stage5/1(din)
  Filt_DEC_by_2_stage4/2(vout) -> Filt_DEC_by_2_stage5/2(vin)
  Filt_DEC_by_2_stage4/3(cout) -> Filt_DEC_by_2_stage5/3(cin)
  Filt_DEC_by_2_stage5/1(dout) -> Filt_DEC_by_2_stage6/1(din)
  Filt_DEC_by_2_stage5/2(vout) -> Filt_DEC_by_2_stage6/2(vin)
  Filt_DEC_by_2_stage5/3(cout) -> Filt_DEC_by_2_stage6/3(cin)

== system Lib_LongPRACH/prach_wrap/FFTShift ==
  data_in : Inport
  data_valid : Inport  Port=2
  chin : Inport  Port=3
  ChNoLatch : Subsystem  Commented=on
  ChannelIn : DSPBAPrim/ChannelIn  primtype=channelin  nInputs=dspba_internal_get_channel_ports(gcb)  nOutputs=dspba_internal_get_channel_ports(gcb)  omode=Inherit via internal rule  otype=sfix(16)  scale=2^-15  rndmethod=Unbiased  factor=1  satmethod=Symmetric  shift_vec=[0 1 2 -1]  value=1  inPortNames=['v'; 'c'; '0'; '1'; '2'; '3'; '4'; '5'; '6'; '7'; '8'; '9'; 'A'; 'B'; 'D'; 'E'; 'F'; 'G'; 'H'; 'I'; 'J'; 'K'; 'L'; 'M'; 'N'; 'O'; 'P'; 'Q'; 'R'; 'S'; 'T'; 'U'; 'W'; 'X'; 'Y'; 'Z']  outPortNames=['v'; 'c'; '0'; '1'; '2'; '3'; '4'; '5'; '6'; '7'; '8'; '9'; 'A'; 'B'; 'D'; 'E'; 'F'; 'G'; 'H'; 'I'; 'J'; 'K'; 'L'; 'M'; 'N'; 'O'; 'P'; 'Q'; 'R'; 'S'; 'T'; 'U'; 'W'; 'X'; 'Y'; 'Z']  dspbaimage=dspba_prim_channel_tall.svg  text=fprintf('In');  style=Optimised  dataSignals=1  foldingEnabled=off  channels=1  sampleRate=200  packetBeginPresent=off  packetBeginEnabled=off  visibilities=dspba_ChannelInVis(gcb)  latencyCorrection=0  scheduleOrigin=on  version=20211214
  ChannelOut : DSPBAPrim/ChannelOut  primtype=channelout  nInputs=dspba_internal_get_channel_ports(gcb)  nOutputs=dspba_internal_get_channel_ports(gcb)  omode=Inherit via internal rule  otype=sfix(16)  scale=2^-15  rndmethod=Unbiased  factor=1  satmethod=Symmetric  shift_vec=[0 1 2 -1]  value=1  inPortNames=['v'; 'c'; '0'; '1'; '2'; '3'; '4'; '5'; '6'; '7'; '8'; '9'; 'A'; 'B'; 'D'; 'E'; 'F'; 'G'; 'H'; 'I'; 'J'; 'K'; 'L'; 'M'; 'N'; 'O'; 'P'; 'Q'; 'R'; 'S'; 'T'; 'U'; 'W'; 'X'; 'Y'; 'Z']  outPortNames=['v'; 'c'; '0'; '1'; '2'; '3'; '4'; '5'; '6'; '7'; '8'; '9'; 'A'; 'B'; 'D'; 'E'; 'F'; 'G'; 'H'; 'I'; 'J'; 'K'; 'L'; 'M'; 'N'; 'O'; 'P'; 'Q'; 'R'; 'S'; 'T'; 'U'; 'W'; 'X'; 'Y'; 'Z']  dspbaimage=dspba_prim_channel_tall.svg  text=fprintf('Out%s', AdvDSPBChannelOutDisplay(latency));  style=Optimised  dataSignals=1  foldingEnabled=off  channels=1  sampleRate=200  packetBeginPresent=off  packetBeginEnabled=off  visibilities=dspba_ChannelOutVis(gcb)  latency=6  latencyCorrection=0  version=20211214
  DualMem : DSPBAPrim/DualMem  primtype=dualmem  nInputs=4  nOutputs=2  omode=Inherit via internal rule  otype=sfix(16)  scale=2^-15  rndmethod=Unbiased  factor=1  satmethod=Symmetric  shift_vec=[0 1 2 -1]  value=[zeros(1024*2, 1)]  inPortNames=['d1'; 'a1'; 'w1'; 'd2'; 'a2'; 'w2']  outPortNames=['q1'; 'q2']  dspbaimage=dspba_prim_tall.svg  text=fprintf('dmem%s',AdvDSPBDMemDisplay(UseDontCare));  style=Optimised  visibilities=8 + 1024 + 2^17 + 2^18  UseDontCare=on  TwinWritePorts=off  init=on  ProvideReadAccess=off  version=20211007
  Mem_rd_wr : Subsystem
  Subsystem : Subsystem
  SynthesisInfo : DSPBAPrim/SynthesisInfo  primtype=synthinfo  nInputs=0  nOutputs=0  omode=Inherit via internal rule  otype=sfix(16)  scale=2^-15  rndmethod=Truncate  factor=1  satmethod=Symmetric  shift_vec=[0 1 2 -1]  value=99  inPortNames=[' '; ' ';]  outPortNames=[' ']  dspbaimage=dspba_prim_ctrl.jpg  text=fprintf('Style=%s', style);  style=Scheduled  visibilities=2^17+2^18+2^19+2^20+2^21+2^22+2^23+2^24  constraintPair=None  constraintRelation=>  constraintLimit=2  modelRefSign=+  modelRef=''  showSchedule=off  simulationMode=Use Global Value  resetMinimization=Conditional - On for ChannelIn/Out only  version=20220106
  Terminator : Terminator
  data_out : Outport
  valid_out : Outport  Port=2
  ch_no : Outport  Port=3
  wires:
  Mem_rd_wr/2(We) -> DualMem/3
  Mem_rd_wr/1(Wr_addr_final) -> DualMem/2
  DualMem/1 -> Terminator/1
  Mem_rd_wr/3(rd_addr_final) -> DualMem/4
  ChannelIn/3 -> DualMem/1
  data_in/1 -> ChannelIn/3
  ChannelIn/1 -> Mem_rd_wr/1(valid)
  data_valid/1 -> ChannelIn/1
  chin/1 -> ChannelIn/2
  ChannelOut/3 -> data_out/1
  DualMem/2 -> ChannelOut/3
  ChannelOut/1 -> valid_out/1
  Mem_rd_wr/4(rd_validout) -> ChannelOut/1
  ChannelOut/2 -> ch_no/1
  Mem_rd_wr/5(wba) -> Subsystem/1(toggleline)
  ChannelIn/2 -> Subsystem/2(d)
  Subsystem/1(q) -> ChannelOut/2

== system Lib_LongPRACH/prach_wrap/MIXER ==
  note: mixer
  din : Inport
  vin : Inport  Port=2
  chin : Inport  Port=3
  sync : Inport  Port=4
  Complex to Real-Imag1 : ComplexToRealImag
  ComplexMixer1 : DSPBAWaveformSynth/ComplexMixer  nInputRate=prach.SampleRateMSPS  nchan=prach.no_of_chan/2  nfreq=NTxAnts  latency=6  simulationMode=Use Global Value  version=20090407
  Const1 : DSPBAPrim/Const  primtype=const  nInputs=0  nOutputs=1  omode=Inherit via back propagation  otype=ufix(8)  scale=2^0  rndmethod=Unbiased  factor=1  satmethod=Symmetric  shift_vec=[0 1 2 -1]  value=1  inPortNames=['+'; '+';]  outPortNames=[' ']  dspbaimage=dspba_prim.svg  text=fprintf('%s', num2str(value));  style=Optimised  visibilities=8 + 1024  floatPrecision=float32_m23  warnSaturation=on  version=20211007  SampleTime=inf
  Const2 : DSPBAPrim/Const  primtype=const  nInputs=0  nOutputs=1  omode=boolean  otype=uint(30)  scale=2^0  rndmethod=Unbiased  factor=1  satmethod=Symmetric  shift_vec=[0 1 2 -1]  value=0  inPortNames=['+'; '+';]  outPortNames=[' ']  dspbaimage=dspba_prim.svg  text=fprintf('%s', num2str(value));  style=Optimised  visibilities=8 + 1024  floatPrecision=float32_m23  warnSaturation=on  version=20211007  SampleTime=inf
  Const6 : DSPBAPrim/Const  primtype=const  nInputs=0  nOutputs=1  omode=Specify via dialog  otype=uint(30)  scale=2^0  rndmethod=Unbiased  factor=1  satmethod=Symmetric  shift_vec=[0 1 2 -1]  value=0  inPortNames=['+'; '+';]  outPortNames=[' ']  dspbaimage=dspba_prim.svg  text=fprintf('%s', num2str(value));  style=Optimised  visibilities=8 + 1024  floatPrecision=float32_m23  warnSaturation=on  version=20211007  SampleTime=inf
  NCO1 : DSPBAWaveformSynth/NCO  outputRate=prach.SampleRateMSPS  otype=sfix(18)  scale=2^-17  accumBitWidth=30  phaseIncrAndInv=ones(1,NTxAnts) *prach.NCO  phaseIncrAndInvMap=MMoffset.NCO  rwmode=Read/Write  exposebus=off  version=20090407  SampleTime=-1  expSFDR=108.36  accumPrecision=+/- 0.05722  phaseIncrInMHz="[48.615  48.615  48.615  48.615]"  outWidth=3  tableSize=8  latency=20
      settings: AttributesFormatString=%<latency>
  Real-Imag to Complex : RealImagToComplex
  Real-Imag to Complex1 : RealImagToComplex
  SampleDelay : DSPBAPrim/SampleDelay  primtype=sampdelay  nInputs=1  nOutputs=1  omode=Inherit via internal rule  otype=sfix(16)  scale=2^-15  rndmethod=Unbiased  factor=1  satmethod=Symmetric  shift_vec=[0 1 2 -1]  floatPrecision=float32_m23  value=1  inPortNames=[' '; ' ';]  outPortNames=[' ']  dspbaimage=dspba_prim.svg  text=dpoly(1, eye(1,value+1), 'z')  style=Optimised  visibilities=8 + 1024 + 2^17 + 2^18  flexible=off  slackgroup=0  augmented=0  version=20211007  advOptions=[]
  SampleDelay1 : DSPBAPrim/SampleDelay  primtype=sampdelay  nInputs=1  nOutputs=1  omode=Inherit via internal rule  otype=sfix(16)  scale=2^-15  rndmethod=Unbiased  factor=1  satmethod=Symmetric  shift_vec=[0 1 2 -1]  floatPrecision=float32_m23  value=1  inPortNames=[' '; ' ';]  outPortNames=[' ']  dspbaimage=dspba_prim.svg  text=dpoly(1, eye(1,value+1), 'z')  style=Optimised  visibilities=8 + 1024 + 2^17 + 2^18  flexible=off  slackgroup=0  augmented=0  version=20211007  advOptions=[]
  Scale : DSPBABase/Scale  otype=sfix(16)  scale=2^-15  rndmethod=Biased  factor=1  satmethod=Symmetric  shift_vec=0  latency=3  simulationMode=Use Global Value  version=20130807
  Scale1 : DSPBABase/Scale  otype=sfix(16)  scale=2^-15  rndmethod=Biased  factor=1  satmethod=Symmetric  shift_vec=0  latency=3  simulationMode=Use Global Value  version=20130807
  Terminator{,1..7} (8 alike) : Terminator
  To Workspace1 : ToWorkspace  VariableName=NCO_valid  SampleTime=-1
  To Workspace5 : ToWorkspace  VariableName=NCO_dout  SampleTime=-1
  delay_FIFO : DSPBAPrim/FIFO  primtype=fifo  nInputs=3  nOutputs=4  omode=Inherit via internal rule  otype=sfix(16)  scale=2^-15  rndmethod=Unbiased  factor=1  satmethod=Symmetric  shift_vec=[0 1 2 -1]  value=[32 4 16]  inPortNames=['w'; 'd'; 'r'; 'f']  outPortNames=['v'; 'q'; 't'; 'f']  dspbaimage=dspba_prim_tall.svg  text=fprintf('fifo');  style=Optimised  visibilities=263168  version=20211007  user_sclr=off
  output4 : Scope  NumInputPorts=5
  dout : Outport  VectorParamsAs1DForOutWhenUnconnected=off
  vout : Outport  Port=2  VectorParamsAs1DForOutWhenUnconnected=off
  cout : Outport  Port=3  VectorParamsAs1DForOutWhenUnconnected=off
  wires:
  Real-Imag to Complex/1 -> dout/1
  Scale/2 -> vout/1
  vin/1 -> delay_FIFO/1, output4/1, SampleDelay/1
  chin/1 -> SampleDelay1/1
  din/1 -> delay_FIFO/2
  Const6/1 -> NCO1/3
  Scale/3 -> cout/1
  delay_FIFO/1 -> Terminator/1
  delay_FIFO/3 -> Terminator2/1
  delay_FIFO/4 -> Terminator1/1
  Scale1/4 -> Terminator3/1
  Scale1/2 -> Terminator5/1
  Scale1/3 -> Terminator6/1
  Scale/1 -> Real-Imag to Complex/1
  Scale1/1 -> Real-Imag to Complex/2
  ComplexMixer1/1 -> Scale/1
  ComplexMixer1/2 -> Scale1/1
  NCO1/2 -> Real-Imag to Complex1/1, output4/5, ComplexMixer1/6
  ComplexMixer1/3 -> Scale1/2, Scale/2
  Complex to Real-Imag1/1 -> ComplexMixer1/1
  NCO1/4 -> output4/3, ComplexMixer1/4
  delay_FIFO/2 -> Complex to Real-Imag1/1
  Complex to Real-Imag1/2 -> ComplexMixer1/2
  Const1/1 -> Scale1/4, Scale/4
  NCO1/1 -> output4/4, ComplexMixer1/5, Real-Imag to Complex1/2
  NCO1/3 -> To Workspace1/1, ComplexMixer1/3, delay_FIFO/3, output4/2
  ComplexMixer1/4 -> Scale1/3, Scale/3
  Scale/4 -> Terminator4/1
  SampleDelay/1 -> NCO1/2
  SampleDelay1/1 -> NCO1/1
  Real-Imag to Complex1/1 -> To Workspace5/1
  sync/1 -> Terminator7/1
  Const2/1 -> NCO1/4
